simulink model "testAlphaWindowIn"  (R2018b)
settings: Solver=VariableStepDiscrete  StartTime=12*3600  StopTime=10+12*3600  MaxStep=1  RelTol=1e-3  EnableMultiTasking=on
libraries: carnot x4, simulink x1
settings Model: Creator=drhf  LastModifiedBy=drhf
settings DataIOCC: LimitDataPoints=on  SaveFormat=Array  ReturnWorkspaceOutputs=on
settings OptimizationCC: DefaultParameterBehavior=Inlined  LifeSpan=inf
settings DebuggingCC: ReadBeforeWriteMsg=DisableAll  WriteAfterWriteMsg=DisableAll  WriteAfterReadMsg=DisableAll  UnderspecifiedInitializationDetection=Classic  MergeDetectMultiDrivingBlocksExec=none  SolverPrmCheckMsg=warning  MultiTaskDSMMsg=none  SFUnexpectedBacktrackingDiag=warning  SFNoUnconditionalDefaultTransitionDiag=warning  SFExecutionAtInitializationDiag=none
settings HardwareCC: ProdBitPerPointer=32  ProdBitPerSizeT=32  ProdBitPerPtrDiffT=32  ProdLargestAtomicFloat=None  ProdIntDivRoundTo=Undefined  ProdEndianess=Unspecified  ProdWordSize=32  ProdHWDeviceType=32-bit Generic
settings ModelReferenceCC: UpdateModelReferenceTargets=IfOutOfDate  PropagateSignalLabelsOutOfModel=off
settings SFSimCC: SFSimEcho=off  SimUseLocalCustomCode=off
settings RTWCC: RTWUseLocalCustomCode=off
settings CodeAppCC: StateflowObjectComments=on
settings GRTTargetCC: TargetLangStandard=C89/C90 (ANSI)  GeneratePreprocessorConditionals=Disable all
settings ConfigComp: CovMetricSettings=dw  CovHtmlReporting=on  CovSaveCumulativeToWorkspaceVar=on  CovSaveSingleToWorkspaceVar=on  CovExternalEMLEnable=off

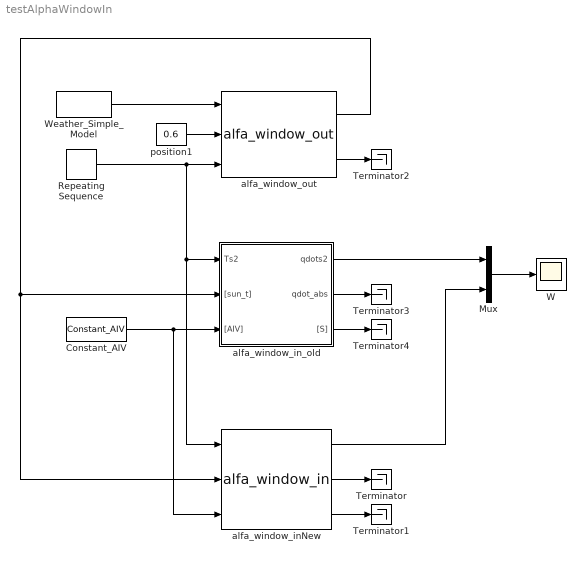
== system testAlphaWindowIn ==
  Constant_AIV : carnot/Source/Ventilation/Constant_AIV  Tsens=20  Tcon=20  Trad=20  mw=0.012  mco=0.01  rhoair=1.2  cpair=1004  pair=100000  nair=0.5
  Mux : Mux  Inputs=2
  Repeating Sequence : simulink/Sources/Repeating Sequence  rep_seq_t=[0 10]  rep_seq_y=[10 30]
  Terminator{,1..4} (5 alike) : Terminator
  W : Scope
  Weather_Simple_Model : carnot/Weather/Weather_Simple_Model  lat=60  Ibn=900  Idg=100  tamb=5  deltaTsky=-6  rh=50  precip="10e-3/24/3600           % 10 mm in 24 h"  cloud=0.125  p=1013e2  vw=1  wdir=270
  alfa_window_inNew : carnot/Basic/Heat_Transfer/alfa_window_in  gvalue=0.7  emission_in=0.87  wallsurface=1  frame=0.1  numlayer=2
  alfa_window_in_old : Subsystem  mask(ALFA){gvalue=0.7, emission_in=0.87, wallsurface=1, frame=0.1, numlayer=2}
      mask prompts: gvalue "Energy transmission by sunlight (g-value) 0..1"; emission_in "Longwave emissivity (0..1)"; wallsurface "Surface of the window (with frame) in m²"; frame "Share of the frame on the surface (0...1)"; numlayer "Number of glass panes"
      mask help:
      | Convective and radiative heat transfer at the INDOOR SURFACE OF A VERTICAL WINDOW with 1-4 layers (each 3 ... 8 mm thick).
      |
      | Ts  : temperature of window surface, °C,
      | [sun_t]  : sun data (incidence angle, direct and diffuse radiation
      |     at tilted window surface),
      | [AIV]  : conditions of zone node,
      | qdots  : specific heat flow into window construction, W/m^2,
      | qdot_abs : specific irradiation absorption within window
      |     construction,  W/m^2,
      | [S]  : heat and air flow to zone node.
  alfa_window_out : carnot/Basic/Heat_Transfer/alfa_window_out  pos=0  absorption_out=0.01  emission_out=0.87  frame=0.1
  position1 : Constant  Value=0.6
  wires:
  Repeating Sequence/1 -> alfa_window_in_old/1(Ts2), alfa_window_inNew/1, alfa_window_out/3
  alfa_window_inNew/1 -> Mux/2
  Mux/1 -> W/1
  Weather_Simple_Model/1 -> alfa_window_out/1
  Constant_AIV/1 -> alfa_window_inNew/3, alfa_window_in_old/3("[AIV]")
  position1/1 -> alfa_window_out/2
  alfa_window_out/1 -> alfa_window_in_old/2("[sun_t]"), alfa_window_inNew/2
  alfa_window_inNew/2 -> Terminator/1
  alfa_window_inNew/3 -> Terminator1/1
  alfa_window_out/2 -> Terminator2/1
  alfa_window_in_old/1(qdots2) -> Mux/1
  alfa_window_in_old/2(qdot_abs) -> Terminator3/1
  alfa_window_in_old/3("[S]") -> Terminator4/1

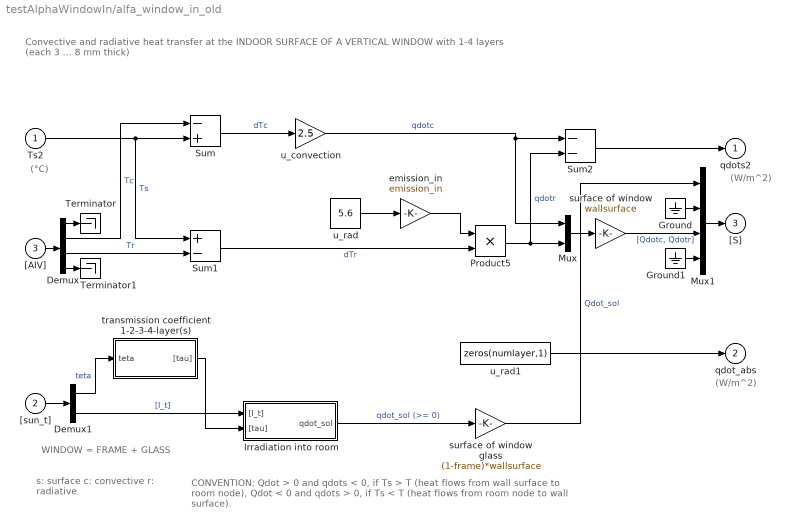
== system testAlphaWindowIn/alfa_window_in_old ==
  note: (W/m^2)
  note: CONVENTION:
      | Qdot > 0 and qdots < 0, if Ts > T (heat flows from wall surface to room node),
      | Qdot < 0 and qdots > 0, if Ts < T (heat flows from room node to wall surface).
  note: s: surface
      | c: convective
      | r: radiative
  note: WINDOW = FRAME + GLASS
  note: (W/m^2)
  note: Convective and radiative heat transfer at the INDOOR SURFACE OF A VERTICAL WINDOW
      | with 1-4 layers (each 3 ... 8 mm thick)
  note: (°C)
  Ts2 : Inport
  "[sun_t]" : Inport  Port=2
  "[AIV]" : Inport  Port=3
  Demux : Demux  Outputs=[1 1 1 6]
  Demux1 : Demux  Outputs=[1 2]
  Ground : Ground
  Ground1 : Ground
  Irradiation into room : Subsystem
  Mux : Mux  Inputs=2
  Mux1 : Mux  Inputs=[1 5 2 5]
  Product5 : Product  SaturateOnIntegerOverflow=on  InputSameDT=on  OutDataTypeStr=Inherit: Same as first input
  Sum : Sum  Inputs=-+  SaturateOnIntegerOverflow=on  InputSameDT=on  OutDataTypeStr=Inherit: Same as first input
  Sum1 : Sum  Inputs=+-  SaturateOnIntegerOverflow=on  InputSameDT=on  OutDataTypeStr=Inherit: Same as first input
  Sum2 : Sum  Inputs=--  SaturateOnIntegerOverflow=on  InputSameDT=on  OutDataTypeStr=Inherit: Same as first input
  Terminator : Terminator
  Terminator1 : Terminator
  emission_in : Gain  Gain=emission_in  SaturateOnIntegerOverflow=on  OutDataTypeStr=Inherit: Same as input  ParamDataTypeStr=Inherit: Same as input
  surface of window : Gain  Gain=wallsurface  SaturateOnIntegerOverflow=on  OutDataTypeStr=Inherit: Same as input  ParamDataTypeStr=Inherit: Same as input
  surface of window glass : Gain  Gain=(1-frame)*wallsurface  SaturateOnIntegerOverflow=on  OutDataTypeStr=Inherit: Same as input  ParamDataTypeStr=Inherit: Same as input
  transmission coefficient 1-2-3-4-layer(s) : Subsystem
  u_convection : Gain  Gain=2.5  SaturateOnIntegerOverflow=on  OutDataTypeStr=Inherit: Same as input  ParamDataTypeStr=Inherit: Same as input
  u_rad : Constant  Value=5.6
  u_rad1 : Constant  Value=zeros(numlayer,1)
  qdots2 : Outport
  qdot_abs : Outport  Port=2
  "[S]" : Outport  Port=3
  wires:
  Ground1/1 -> Mux1/4
  Ground/1 -> Mux1/2
  Mux1/1 -> "[S]"/1
  Sum2/1 -> qdots2/1
  Demux/4 -> Terminator1/1
  "[AIV]"/1 -> Demux/1
  Demux/1 -> Terminator/1
  Mux/1 -> surface of window/1
  emission_in/1 -> Product5/1
  Sum1/1 -> Product5/2  "dTr"
  u_rad/1 -> emission_in/1
  Ts2/1 -> Sum/2, Sum1/1  "Ts"
  Product5/1 -> Mux/2, Sum2/2  "qdotr"
  u_convection/1 -> Sum2/1, Mux/1  "qdotc"
  Irradiation into room/1(qdot_sol) -> surface of window glass/1  "qdot_sol (>= 0)"
  Demux1/1 -> transmission coefficient 1-2-3-4-layer(s)/1(teta)  "teta"
  "[sun_t]"/1 -> Demux1/1
  surface of window glass/1 -> Mux1/1  "Qdot_sol"
  surface of window/1 -> Mux1/3  "[Qdotc, Qdotr]"
  Demux/2 -> Sum/1  "Tc"
  u_rad1/1 -> qdot_abs/1
  Sum/1 -> u_convection/1  "dTc"
  Demux/3 -> Sum1/2  "Tr"
  Demux1/2 -> Irradiation into room/1("[I_t]")  "[I_t]"
  transmission coefficient 1-2-3-4-layer(s)/1("[tau]") -> Irradiation into room/2("[tau]")

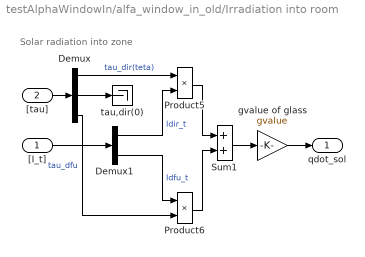
== system testAlphaWindowIn/alfa_window_in_old/Irradiation into room ==
  note: Solar radiation into zone
  "[I_t]" : Inport
  "[tau]" : Inport  Port=2
  Demux : Demux  Outputs=3
  Demux1 : Demux  Outputs=2
  Product5 : Product  SaturateOnIntegerOverflow=on  InputSameDT=on  OutDataTypeStr=Inherit: Same as first input
  Product6 : Product  SaturateOnIntegerOverflow=on  InputSameDT=on  OutDataTypeStr=Inherit: Same as first input
  Sum1 : Sum  SaturateOnIntegerOverflow=on  InputSameDT=on  OutDataTypeStr=Inherit: Same as first input
  gvalue of glass : Gain  Gain=gvalue  SaturateOnIntegerOverflow=on  OutDataTypeStr=Inherit: Same as input  ParamDataTypeStr=Inherit: Same as input
  tau,dir(0) : Terminator
  qdot_sol : Outport
  wires:
  gvalue of glass/1 -> qdot_sol/1
  Sum1/1 -> gvalue of glass/1
  "[tau]"/1 -> Demux/1
  Demux/1 -> Product5/1  "tau_dir(teta)"
  Demux/2 -> tau,dir(0)/1
  "[I_t]"/1 -> Demux1/1
  Demux1/2 -> Product6/1  "Idfu_t"
  Demux1/1 -> Product5/2  "Idir_t"
  Demux/3 -> Product6/2  "tau_dfu"
  Product6/1 -> Sum1/2
  Product5/1 -> Sum1/1

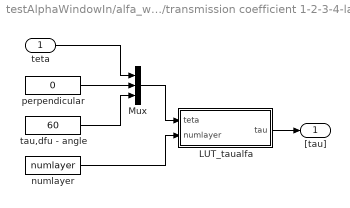
== system testAlphaWindowIn/alfa_window_in_old/transmission coefficient 1-2-3-4-layer(s) ==
  teta : Inport
  LUT_taualfa : Subsystem  mask(LOOK UP TABLE){}
      mask help:
      | This block delivers the standardized LIGHT TRANSMISSION COEFFICIENT of a window glass with 1, 2, 3 or 4 layers depending on the incidence angle. Each layer may be 3 to 8 mm thick.
      |
      | teta:    incidence angle = angle between surface normal and
      |                 incidence, degree
      | numlayer: number of layers within the window glass, [1,4].
      | tau:    transmission of glass layer stack, [0,1]
  Mux : Mux  Inputs=3
  numlayer : Constant  Value=numlayer
  perpendicular : Constant  Value=0
  tau,dfu - angle : Constant  Value=60
  "[tau]" : Outport
  wires:
  LUT_taualfa/1(tau) -> "[tau]"/1
  numlayer/1 -> LUT_taualfa/2(numlayer)
  Mux/1 -> LUT_taualfa/1(teta)
  perpendicular/1 -> Mux/2
  tau,dfu - angle/1 -> Mux/3
  teta/1 -> Mux/1

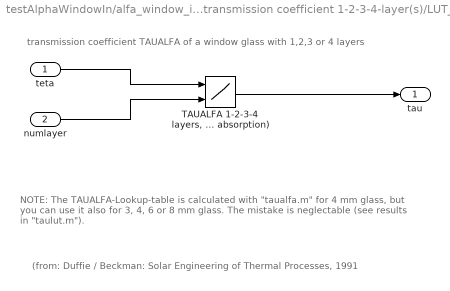
== system testAlphaWindowIn/alfa_window_in_old/transmission coefficient 1-2-3-4-layer(s)/LUT_taualfa ==
  note: NOTE: The TAUALFA-Lookup-table is calculated with "taualfa.m"
      | for 4 mm glass, but you can use it also for  3, 4, 6 or 8 mm glass.
      | The mistake is neglectable (see results in "taulut.m").
  note: transmission coefficient TAUALFA of a window glass with 1,2,3 or 4 layers
  note: (from: Duffie / Beckman: Solar Engineering of Thermal Processes, 1991
  teta : Inport
  numlayer : Inport  Port=2
  "TAUALFA 1-2-3-4 layers, standardized to 1.0, (4 mm float glass, no dirt absorption, 97% room absorption)" : Lookup2D  RowIndex=[0:10:90]  ColumnIndex=[1:4]  Table=[1.0000 1.0000 1.0000 1.0000; 0.9996 0.9991 0.9987 0.9983; 0.9979 0.9961 0.9945 0.9929; 0.9937 0.9894 0.9861 0.9836; 0.9839 0.9753 0.9704 0.9680; 0.9608 0.9438 0.9365 0.9361; 0.9061 0.8679 0.8484 0.8413; 0.7755 0.6821 0.6182 0.5717; 0.4807 0.3277 0.2324 0.1688; 0 0 0 0]  SaturateOnIntegerOverflow=on  InputSameDT=on
  tau : Outport
  wires:
  teta/1 -> "TAUALFA 1-2-3-4 layers, standardized to 1.0, (4 mm float glass, no dirt absorption, 97% room absorption)"/1
  numlayer/1 -> "TAUALFA 1-2-3-4 layers, standardized to 1.0, (4 mm float glass, no dirt absorption, 97% room absorption)"/2
  "TAUALFA 1-2-3-4 layers, standardized to 1.0, (4 mm float glass, no dirt absorption, 97% room absorption)"/1 -> tau/1
